simulink model "celp_sq"  (Simulink 6.1)
settings: Solver=FixedStepDiscrete  SolverMode=SingleTasking  StartTime=0.0  StopTime=3  RelTol=1e-3
PreLoadFcn:
  | load lpcvocoder.mat;
undefined symbols (not defined in the file): jet, magnitude, poly2lsf
libraries: simulink x25, dspindex x17, dspcelplib x14, dsparch4 x12, dspquant2 x10, dspstat3 x10, dspsrcs4 x9, dspbuff3 x8, dspsigops x7, dspmtrx3 x6, dsplp x5, dspmathops x4
(part 2 of 2)

== system celp_sq/CELP Decoder/Subframe Synthesis/Formant Post Filter/Subsystem for ARMA Coefficients ==
  Lpc : Inport  Port=1  LatchInput=off
  Bandwidth Expansion : Subsystem  mask(Bandwidth Expansion){alpha=0.65}
      mask prompts: alpha "Bandwidth expansion factor:"
      mask help:
      | Generate autoregressive (AR) polynomial with bandwidth expanded relative to the bandwidth of the input AR polynomial.
      |
      | By reducing the radius of the roots in an autoregressive polynomial (i.e., scaling them towards the origin of the Z-plane), the bandwidth of the spectral peaks in the frequency response is expanded (flattened).  This operation is often referred to as "bandwidth expansion".
      |
      | Bandwidth expansion factor must be in the range [0,1], where 1.0 yields no changes to the roots of the polynomial.
      mask Help: web(dspbhelp);
      mask Display: fprintf('Bandwidth\nExpansion\n%g', alpha)
  Bandwidth Expansion1 : Subsystem  mask(Bandwidth Expansion){alpha=0.75}
      mask prompts: alpha "Bandwidth expansion factor:"
      mask help:
      | Generate autoregressive (AR) polynomial with bandwidth expanded relative to the bandwidth of the input AR polynomial.
      |
      | By reducing the radius of the roots in an autoregressive polynomial (i.e., scaling them towards the origin of the Z-plane), the bandwidth of the spectral peaks in the frequency response is expanded (flattened).  This operation is often referred to as "bandwidth expansion".
      |
      | Bandwidth expansion factor must be in the range [0,1], where 1.0 yields no changes to the roots of the polynomial.
      mask Help: web(dspbhelp);
      mask Display: fprintf('Bandwidth\nExpansion\n%g', alpha)
  FirCoef : Outport
  IirCoef : Outport  Port=2
  wires:
  Lpc/1 -> Bandwidth Expansion/1(In1), Bandwidth Expansion1/1(In1)
  Bandwidth Expansion1/1(Out1) -> IirCoef/1
  Bandwidth Expansion/1(Out1) -> FirCoef/1

== system celp_sq/CELP Decoder/Subframe Synthesis/Gain Scaling Unit/For Iterator Subsystem1 ==
  note: g(n)
  note: y(n)
  note: y(n)=g(n)+0.9375y(n-1)
      | with IC=1
  note: Computation of gain scaling factor for each sample of the subframe
  ScalarGain : Inport  Port=1  LatchInput=off
  Assignment : Assignment  ElementSrc=External  Rows=-1  ColumnSrc=External
  Constant1 : Constant  Orientation=down  Value=zeros(40,1)  VectorParams1D=off
  For Iterator : ForIterator  IterationLimit=40
  filter : dsparch4/Digital Filter  DialogController=dspDDGCreate  DialogControllerArgs=DataTag8  TypePopup=IIR (all poles)  IIRFiltStruct=Direct form II transposed  AllPoleFiltStruct=Direct form  FIRFiltStruct=Direct form  CoeffSource=Specify via dialog  NumCoeffs=[1 -.95]  DenCoeffs="[1   -0.9375]"  BiQuadCoeffs=[1 0.3 0.4 1 0.1 0.2]  LatticeCoeffs=[0.2 0.4]  denIgnore=on  FiltPerSampPopup=One filter per frame  IC=1  ICnum=0  ICden=0  roundingMode=Floor  overflowMode=off  ScaleValues=1  scaleValueFracLength=14  stageInFracLength=15  stageOutFracLength=15
  VectorGain : Outport
  wires:
  For Iterator/1 -> Assignment/3
  Assignment/1 -> VectorGain/1
  Constant1/1 -> Assignment/1
  ScalarGain/1 -> filter/1
  filter/1 -> Assignment/2

== system celp_sq/CELP Decoder/Subframe Synthesis/Reconstruction of  Speech Subframe/Harmonic Shaper ==
  inRes : Inport  Port=1  LatchInput=off
  Delay : Inport  Port=2  LatchInput=off
  Beta : Inport  Port=3  LatchInput=off
  1-bz^(-D)2 : Subsystem  TreatAsAtomicUnit=on
  Energy normalization : Subsystem
  Pitch Synthesis Filtering 1/(1-b.z^(-D))2 : dsparch4/Digital Filter  DialogController=dspDDGCreate  DialogControllerArgs=DataTag9  TypePopup=IIR (all poles)  IIRFiltStruct=Direct form II transposed  AllPoleFiltStruct=Direct form  FIRFiltStruct=Direct form  CoeffSource=Input port(s)  NumCoeffs=[1 -.95]  DenCoeffs=[1 0.1]  BiQuadCoeffs=[1 0.3 0.4 1 0.1 0.2]  LatticeCoeffs=[0.2 0.4]  denIgnore=on  FiltPerSampPopup=One filter per frame  IC=0  ICnum=0  ICden=0  roundingMode=Floor  overflowMode=off  ScaleValues=1  scaleValueFracLength=14  stageInFracLength=15  stageOutFracLength=15
  OutRes : Outport
  wires:
  Pitch Synthesis Filtering 1/(1-b.z^(-D))2/1 -> Energy normalization/2(SigNew)
  inRes/1 -> Energy normalization/1(SigOrg), Pitch Synthesis Filtering 1/(1-b.z^(-D))2/1
  1-bz^(-D)2/1(Polynom) -> Pitch Synthesis Filtering 1/(1-b.z^(-D))2/2
  Delay/1 -> 1-bz^(-D)2/1(D_buf_1based)
  Beta/1 -> 1-bz^(-D)2/2(beta)
  Energy normalization/1(SigNew2) -> OutRes/1  "res"

== system celp_sq/CELP Decoder/Subframe Synthesis/Reconstruction of  Speech Subframe/LP Synthesis Filter ==
  Residual : Inport  Port=1  LatchInput=off
  LSF : Inport  Port=2  LatchInput=off
  LPC to/from RC : dsplp/LPC to//from RC  conversion=LPC to RC  perr=off  stability=off  error=Replace it with 1
  LSF/LSP to LPC Conversion : dsplp/LSF//LSP to LPC Conversion  input=LSF in range (0 pi)
  Time-Varying  Synthesis Filter 1/A(z) : dsparch4/Digital Filter  DialogController=dspDDGCreate  DialogControllerArgs=DataTag10  TypePopup=IIR (all poles)  IIRFiltStruct=Direct form II transposed  AllPoleFiltStruct=Lattice AR  FIRFiltStruct=Direct form  CoeffSource=Input port(s)  NumCoeffs=[1 -.95]  DenCoeffs=[1 0.1]  BiQuadCoeffs=[1 0.3 0.4 1 0.1 0.2]  LatticeCoeffs=[0.2 0.4]  denIgnore=off  FiltPerSampPopup=One filter per frame  IC=0  ICnum=0  ICden=0  roundingMode=Floor  overflowMode=off  ScaleValues=1  scaleValueFracLength=14  stageInFracLength=15  stageOutFracLength=15
  Sig : Outport
  LPC : Outport  Port=2
  wires:
  LSF/LSP to LPC Conversion/1 -> LPC to/from RC/1, LPC/1
  LPC to/from RC/1 -> Time-Varying  Synthesis Filter 1/A(z)/2
  Residual/1 -> Time-Varying  Synthesis Filter 1/A(z)/1
  Time-Varying  Synthesis Filter 1/A(z)/1 -> Sig/1  "S(n)"
  LSF/1 -> LSF/LSP to LPC Conversion/1

== system celp_sq/CELP Decoder/Subframe Synthesis/Reconstruction of  Speech Subframe/Pitch synthesis ==
  PitchRes : Inport  Port=1  LatchInput=off
  Delay : Inport  Port=2  LatchInput=off
  Beta : Inport  Port=3  LatchInput=off
  1-bz^(-D) : Subsystem  TreatAsAtomicUnit=on
  Pitch synthesis Filter 1/(1-b.z^(-D)) : dsparch4/Digital Filter  DialogController=dspDDGCreate  DialogControllerArgs=DataTag11  TypePopup=IIR (all poles)  IIRFiltStruct=Direct form II transposed  AllPoleFiltStruct=Direct form  FIRFiltStruct=Direct form  CoeffSource=Input port(s)  NumCoeffs=[1 -.95]  DenCoeffs=[1 0.1]  BiQuadCoeffs=[1 0.3 0.4 1 0.1 0.2]  LatticeCoeffs=[0.2 0.4]  denIgnore=on  FiltPerSampPopup=One filter per frame  IC=0  ICnum=0  ICden=0  roundingMode=Floor  overflowMode=off  ScaleValues=1  scaleValueFracLength=14  stageInFracLength=15  stageOutFracLength=15
  LPRes : Outport
  wires:
  1-bz^(-D)/1(Polynom) -> Pitch synthesis Filter 1/(1-b.z^(-D))/2
  Delay/1 -> 1-bz^(-D)/1(D_buf_1based)
  Beta/1 -> 1-bz^(-D)/2(beta)
  PitchRes/1 -> Pitch synthesis Filter 1/(1-b.z^(-D))/1
  Pitch synthesis Filter 1/(1-b.z^(-D))/1 -> LPRes/1

== system celp_sq/CELP Decoder/Subframe Synthesis/Reconstruction of  Speech Subframe/Reconstruction of  Pitch Residual Signal ==
  4SignBit : Inport  Port=1  LatchInput=off
  4Position : Inport  Port=2  LatchInput=off
  FCBgain : Inport  Port=3  LatchInput=off
  Frame Status : FrameConversion  OutFrame=Sample based
  Frame Status1 : FrameConversion  OutFrame=Sample based
  Product4 : Product  OutDataTypeMode=double  SaturateOnIntegerOverflow=on
  replace 4 selected samples by their sign and set others to zero : Subsystem  TreatAsAtomicUnit=on
  qPitchRes : Outport
  wires:
  Frame Status/1 -> replace 4 selected samples by their sign and set others to zero/1(4SignBit)
  Frame Status1/1 -> replace 4 selected samples by their sign and set others to zero/2(4Position)
  replace 4 selected samples by their sign and set others to zero/1(newPitchRes) -> Product4/1
  4SignBit/1 -> Frame Status/1
  4Position/1 -> Frame Status1/1
  Product4/1 -> qPitchRes/1
  FCBgain/1 -> Product4/2

== system celp_sq/CELP Encoder/Frame Analysis/Classical LPC analysis/  ==
  note: In this subsystem, LPC analysis is performed on a speech signal with a
      |
      | frame size of 30 ms (240 samples). This signal has an overlap of 10 ms
      |
      | (80 samples). Each frame is windowed using a Hamming window and 10th order
      |
      | autocorrelation coefficients are found. Using the Levinson Durbin
      |
      | algorithm, 10th order LP coefficients are calculated from the
      |
      | autocorrelation coefficients. Finally, the LP coefficients are modified
      |
      | using a bandwidth expansion block.

== system celp_sq/CELP Encoder/Frame Analysis/Classical LPC analysis/Bandwidth Expansion ==
  In1 : Inport  Port=1  LatchInput=off
  Window Function : dspsigops/Window Function  DialogController=dspDDGCreate  DialogControllerArgs=DataTag14  winmode=Apply window to input  wintype=User defined  sampmode=Continuous  samptime=1  N=64  Rs=50  beta=10  winsamp=Symmetric  UserWindow=bwexpwin  OptParams=on  UserParams=alpha  dataType=double  isSigned=on  wordLen=16  udDataType=sfix(16)  fracBitsMode=Best precision  numFracBits=15  roundingMode=Floor  overflowMode=off
  Out1 : Outport
  wires:
  In1/1 -> Window Function/1
  Window Function/1 -> Out1/1

== system celp_sq/CELP Encoder/Frame Analysis/LSF Interpolation/  ==
  note: In this subsystem the LSFs are interpolated, in order to:
      |
      | 1.  Avoid rapid changes in the LP parameters (LSFs) between successive frames
      |
      | 2.  Specify the synthesis filter parameters for each subframe.

== system celp_sq/CELP Encoder/Frame Analysis/LSF Vector Quantization/  ==
  note: In this portion of the subsystems, the following operations occur:
      |
      |
      | 1. Linear prediction (LP) coefficients are converted to line spectral
      |
      |    frequencies (LSFs). After quantization and interpolation, the stability
      |
      |    of the LP synthesis filter can be guaranteed in the LSF domain without
      |
      |    additional computation.
      |
      |
      | 2. Weighting factors used in the LSF quantization are calculated using the
      |
      |    method proposed by Paliwal and Atal*. In this method, the weight
      |
      |    assigned to a given LSF is proportional to the spectral sensitivity and
      |
      |    the value of the spectral envelope at the current LSF.
      |
      | *[ K.K. Paliwal and B.S. Atal, "Efficient vector quantization of LPC
      |
      |    parameters at 24 bits/frame," J. Acoust. Soc. Am., vol. 87, p. S39, 1990]

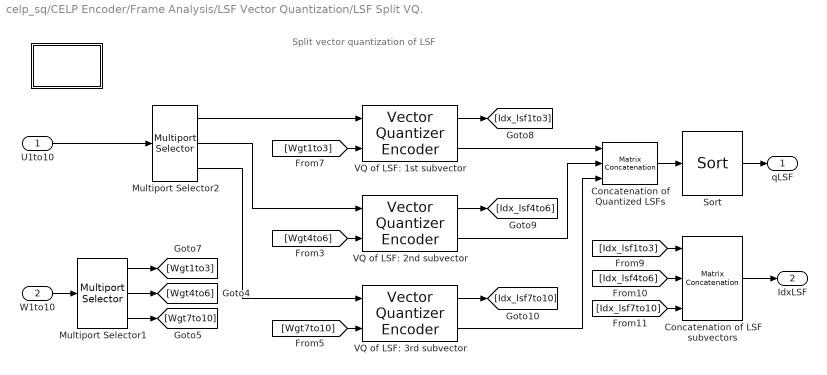
== system celp_sq/CELP Encoder/Frame Analysis/LSF Vector Quantization/LSF Split VQ. ==
  note: Split vector quantization of LSF
  U1to10 : Inport  Port=1  LatchInput=off
  W1to10 : Inport  Port=2  LatchInput=off
  " " : Subsystem
      mask Type: CELP Coder Demo Info
      mask Display: disp('Info')
  Concatenation of LSF subvectors : simulink/Math Operations/Matrix Concatenation  numInports=3  catMethod=Horizontal
  Concatenation of Quantized LSFs : simulink/Math Operations/Matrix Concatenation  numInports=3  catMethod=Vertical
  Multiport Selector1 : dspindex/Multiport Selector  rowsOrCols=Rows  idxCellArray={1:3,4:6,7:10}  idxErrMode=Clip Index
  Multiport Selector2 : dspindex/Multiport Selector  rowsOrCols=Rows  idxCellArray={1:3,4:6,7:10}  idxErrMode=Clip Index
  Sort : dspstat3/Sort  DialogController=dspDDGCreate  DialogControllerArgs=DataTag17  otype=Value  dir=Ascending  sortAlg=Quick sort  roundingMode=Floor  overflowMode=off
  VQ of LSF: 1st subvector : dspquant2/Vector Quantizer Encoder  CBsource=Specify via dialog  codebook=CB_lsf1to3_10bit  distMeasure=Weighted squared error  wgtSrc=Input port  weights=[1 1 1]  tieBreakRule=Choose the lower index  outQU=on  outQError=off  idtype=int32  roundingMode=Floor  overflowMode=off
  VQ of LSF: 2nd subvector : dspquant2/Vector Quantizer Encoder  CBsource=Specify via dialog  codebook=CB_lsf4to6_10bit  distMeasure=Weighted squared error  wgtSrc=Input port  weights=[1 1 1]  tieBreakRule=Choose the lower index  outQU=on  outQError=off  idtype=int32  roundingMode=Floor  overflowMode=off
  VQ of LSF: 3rd subvector : dspquant2/Vector Quantizer Encoder  CBsource=Specify via dialog  codebook=CB_lsf7to10_10bit  distMeasure=Weighted squared error  wgtSrc=Input port  weights=[1 1 1]  tieBreakRule=Choose the lower index  outQU=on  outQError=off  idtype=int32  roundingMode=Floor  overflowMode=off
  qLSF : Outport
  IdxLSF : Outport  Port=2
  wires:
  VQ of LSF: 1st subvector/2 -> Concatenation of Quantized LSFs/1
  VQ of LSF: 1st subvector/1 -> [Idx_lsf1to3]
  Multiport Selector2/2 -> VQ of LSF: 2nd subvector/1
  Multiport Selector2/3 -> VQ of LSF: 3rd subvector/1
  Multiport Selector1/2 -> [Wgt4to6]
  Multiport Selector1/3 -> [Wgt7to10]
  VQ of LSF: 2nd subvector/1 -> [Idx_lsf4to6]
  [Wgt7to10] -> VQ of LSF: 3rd subvector/2
  VQ of LSF: 3rd subvector/1 -> [Idx_lsf7to10]
  VQ of LSF: 2nd subvector/2 -> Concatenation of Quantized LSFs/2
  Concatenation of Quantized LSFs/1 -> Sort/1
  VQ of LSF: 3rd subvector/2 -> Concatenation of Quantized LSFs/3
  [Wgt4to6] -> VQ of LSF: 2nd subvector/2
  Multiport Selector1/1 -> [Wgt1to3]
  [Wgt1to3] -> VQ of LSF: 1st subvector/2
  [Idx_lsf1to3] -> Concatenation of LSF subvectors/1
  [Idx_lsf4to6] -> Concatenation of LSF subvectors/2
  [Idx_lsf7to10] -> Concatenation of LSF subvectors/3
  W1to10/1 -> Multiport Selector1/1
  U1to10/1 -> Multiport Selector2/1
  Sort/1 -> qLSF/1
  Concatenation of LSF subvectors/1 -> IdxLSF/1
  Multiport Selector2/1 -> VQ of LSF: 1st subvector/1

== system celp_sq/CELP Encoder/Frame Analysis/LSF Vector Quantization/Paliwal Weight  Computation ==
  note: Calculation of Perceptual Weighting Factors
  LSF : Inport  Port=1  LatchInput=off
  LPC : Inport  Port=2  LatchInput=off
  " " : Subsystem
      mask Type: CELP Coder Demo Info
      mask Display: disp('Info')
  Constant : Constant  Orientation=up  Value=0.15  VectorParams1D=off  SampleTime=-1
  Gain : Gain  Gain=-1
  Gain1 : Gain  Gain=[ones(1,8) 0.8 0.4]
  LPCpowSpec : Subsystem
  Math Function : Math  Operator=pow  SaturateOnIntegerOverflow=on
  Reshape : simulink/Math Operations/Reshape  OutputDimensionality=Column vector  OutputDimensions=[1,1]
  Submatrix : dspmtrx3/Submatrix  RowSpan=Range of rows  RowStartMode=Index  RowStartIndex=2  RowEndMode=Last  RowEndIndex=1  ColSpan=All columns  ColStartMode=First  ColStartIndex=1  ColEndMode=Last  ColEndIndex=1
  Weights : Outport
  wires:
  LPCpowSpec/1(Out) -> Math Function/1
  Constant/1 -> Math Function/2
  Math Function/1 -> Gain1/1
  Gain1/1 -> Reshape/1
  LSF/1 -> LPCpowSpec/2(LSF)
  Reshape/1 -> Weights/1
  Submatrix/1 -> Gain/1
  LPC/1 -> Submatrix/1
  Gain/1 -> LPCpowSpec/1(PC)

== system celp_sq/CELP Encoder/Subframe Analysis/Innovation signal quantization/  ==
  note: In this subsystem, the four "most significant pulses" are found from a
      |
      | subframe of length 40. Also, FCB gain is computed.
      |
      |
      |
      | 1. The absolute values of the 40 subframe samples are sorted in descending
      |
      | order. Their original positions are stored in a variable that has the
      |
      | following format: pos = [pos1, pos2, ..., pos40]. Here, pos1 stores the
      |
      | position of the largest valued sample, pos2 stores the position of the
      |
      | second largest valued sample, and so on.
      |
      |
      | 2.  The first four dominant samples are replaced by a +1 or a -1, where +1
      |
      | represents a positive sample and  -1 represents a negative sample. The
      |
      | other 36 samples are replaced by zeros. For example, a +1 or a -1 would be
      |
      | located at positions pos1, pos2, pos3, and pos4, and zeros would occupy the
      |
      | other positions.
      |
      |
      | 3. The zero-state response of the synthesis filter 1/A(z) to the original
      |
      | pitch residual signal is computed.
      |
      | 4. The zero-state response of the synthesis filter 1/A(z) to the quantized
      |
      | pitch residual signal is computed using the method of sparse filtering.
      |
      | Here, first the impulse response of the filter is calculated. Then the
      |
      | impulse response is convolved with the sparse representation of the
      |
      | quantized pitch residual signal.
      |
      |
      | 5. Steps 2 and 4 are repeated with four new samples from positions pos2,
      |
      | pos3, pos4, and pos5.
      |
      |
      |
      | This process is repeated for all 37 combinations of the positions. The set
      |
      | of four positions that minimize the error between the zero state response
      |
      | to the original pitch residual signal and the zero state response to the
      |
      | quantized pitch residual are the four "most significant pulses".

== system celp_sq/CELP Encoder/Subframe Analysis/Innovation signal quantization/Impulse Response ==
  In1 : Inport  Port=1  LatchInput=off
  DSP Constant : dspsrcs4/DSP Constant  Value=[1;zeros(39,1)]  SampleMode=Discrete  discreteOutput=Frame-based  continuousOutput=Sample-based  sampTime=1  framePeriod=-1  dataType=Inherit from 'Constant value'  isSigned=on  wordLen=16  udDataType=sfix(16)  fracBitsMode=Best precision  numFracBits=15  InterpretAs1D=-inf  Ts=-inf  FramebasedOutput=-inf
  For Iterator Subsystem2 : Subsystem  TreatAsAtomicUnit=on
      mask Display:
      | disp('Zero State\nIIR Lattice\nFilter');
      | port_label('input',1,'In');
      | port_label('input',2,'K');
      | port_label('output',1,'Out');
  Out1 : Outport
  wires:
  For Iterator Subsystem2/1(SigOut2) -> Out1/1
  In1/1 -> For Iterator Subsystem2/2(K)
  DSP Constant/1 -> For Iterator Subsystem2/1(SigIn2)

== system celp_sq/CELP Encoder/Subframe Analysis/Innovation signal quantization/Searching for FCB pulse  positions and FCB gain ==
  note: To Search for FCB pulse positions and FCB gain
  PitchRes : Inport  Port=1  LatchInput=off
  Idx : Inport  Port=2  LatchInput=off
  e_n : Inport  Port=3  LatchInput=off
  h : Inport  Port=4  LatchInput=off
  " " : Subsystem
      mask Type: CELP Coder Demo Info
      mask Display: disp('Info')
  1-based to  0-based : Bias  Bias=-1
  Computation of  Error and Gain : Subsystem
  For Iterator : ForIterator  ResetStates=reset  IterationLimit=37
  Optimal Features : Subsystem
  Partial decomposition of  Pitch Residual : Subsystem
  Signal to sign bit : Subsystem
  pos_sign_g : Outport
  wires:
  1-based to  0-based/1 -> Computation of  Error and Gain/2(4Pos)
  h/1 -> Computation of  Error and Gain/4(h)
  e_n/1 -> Computation of  Error and Gain/3(e_n)
  Signal to sign bit/1(SignBit) -> Computation of  Error and Gain/1(4Val), Optimal Features/1(SignBit)
  Partial decomposition of  Pitch Residual/2(4Idx) -> 1-based to  0-based/1, Optimal Features/4(Pos)
  Partial decomposition of  Pitch Residual/1(4Val) -> Signal to sign bit/1(Sig)
  For Iterator/1 -> Partial decomposition of  Pitch Residual/3(Control)
  Idx/1 -> Partial decomposition of  Pitch Residual/2(Idx)
  PitchRes/1 -> Partial decomposition of  Pitch Residual/1(PitchRes)
  Computation of  Error and Gain/1(Err) -> Optimal Features/2(Err)
  Computation of  Error and Gain/2(G) -> Optimal Features/3(G)
  Optimal Features/1(Features) -> pos_sign_g/1

== system celp_sq/CELP Encoder/Subframe Analysis/Innovation signal quantization/filter ==
  SigIn2 : Inport  Port=1  LatchInput=off
  K : Inport  Port=2  LatchInput=off
  " " : Subsystem
      mask Type: CELP Coder Demo Info
      mask Display: disp('Info')
  For Iterator : ForIterator  ResetStates=reset  IterationLimit=1  ShowIterationPort=off
  Time-Varying  Synthesis Filter 1/A(z). : dsparch4/Digital Filter  DialogController=dspDDGCreate  DialogControllerArgs=DataTag22  TypePopup=IIR (all poles)  IIRFiltStruct=Direct form II transposed  AllPoleFiltStruct=Lattice AR  FIRFiltStruct=Direct form  CoeffSource=Input port(s)  NumCoeffs=[1 -.95]  DenCoeffs=[1 0.1]  BiQuadCoeffs=[1 0.3 0.4 1 0.1 0.2]  LatticeCoeffs=[0.2 0.4]  denIgnore=off  FiltPerSampPopup=One filter per frame  IC=0  ICnum=0  ICden=0  roundingMode=Floor  overflowMode=off  ScaleValues=1  scaleValueFracLength=14  stageInFracLength=15  stageOutFracLength=15
  SigOut2 : Outport
  wires:
  Time-Varying  Synthesis Filter 1/A(z)./1 -> SigOut2/1
  SigIn2/1 -> Time-Varying  Synthesis Filter 1/A(z)./1
  K/1 -> Time-Varying  Synthesis Filter 1/A(z)./2

== system celp_sq/CELP Encoder/Subframe Analysis/Pitch Estimation/  ==
  note: Here the following operations occur:
      |
      | 1. The LPC residual signal is obtained by filtering the speech by the
      |     quantized and interpolated LPC analysis filter, A(Z).
      |
      | 2. The parameters specifying the adaptive component of the excitation
      |     (pitch lag and pitch gain) are computed using the open loop pitch estimation
      |     by minimizing the error between the current residual signal and its
      |     scaled-and-delayed version.

== system celp_sq/CELP Encoder/Subframe Analysis/Pitch Estimation/LPC Residual Calculation ==
  Speech : Inport  Port=1  LatchInput=off
  LSF : Inport  Port=2  LatchInput=off
  LPC to/from RC : dsplp/LPC to//from RC  conversion=LPC to RC  perr=off  stability=off  error=Replace it with 1
  LSF/LSP to LPC Conversion : dsplp/LSF//LSP to LPC Conversion  input=LSF in range (0 pi)
  Time-Varying  Analysis Filter A(z) : dsparch4/Digital Filter  DialogController=dspDDGCreate  DialogControllerArgs=DataTag23  TypePopup=FIR (all zeros)  IIRFiltStruct=Direct form II transposed  AllPoleFiltStruct=Direct form  FIRFiltStruct=Lattice MA  CoeffSource=Input port(s)  NumCoeffs=[1 -.95]  DenCoeffs=[1 0.1]  BiQuadCoeffs=[1 0.3 0.4 1 0.1 0.2]  LatticeCoeffs=[0.2 0.4]  denIgnore=on  FiltPerSampPopup=One filter per frame  IC=0  ICnum=0  ICden=0  roundingMode=Floor  overflowMode=off  ScaleValues=1  scaleValueFracLength=14  stageInFracLength=15  stageOutFracLength=15
  Residual : Outport
  K : Outport  Port=2
  wires:
  LSF/LSP to LPC Conversion/1 -> LPC to/from RC/1
  Speech/1 -> Time-Varying  Analysis Filter A(z)/1
  Time-Varying  Analysis Filter A(z)/1 -> Residual/1
  LSF/1 -> LSF/LSP to LPC Conversion/1
  LPC to/from RC/1 -> Time-Varying  Analysis Filter A(z)/2, K/1

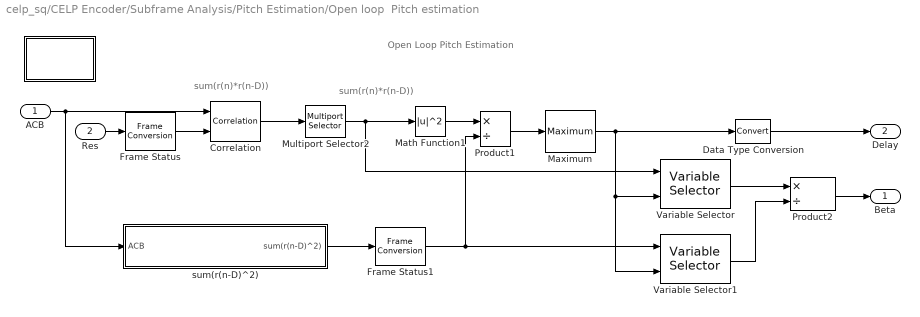
== system celp_sq/CELP Encoder/Subframe Analysis/Pitch Estimation/Open loop  Pitch estimation ==
  note: sum(r(n)*r(n-D))
  note: sum(r(n)*r(n-D))
  note: Open Loop Pitch Estimation
  ACB : Inport  Port=1  LatchInput=off
  Res : Inport  Port=2  LatchInput=off
  " " : Subsystem
      mask Type: CELP Coder Demo Info
      mask Display: disp('Info')
  Correlation : dspstat3/Correlation  DialogController=dspDDGCreate  DialogControllerArgs=DataTag24  domain=Fastest  roundingMode=Floor  overflowMode=off
  Data Type Conversion : DataTypeConversion  OutDataTypeMode=int32  SaturateOnIntegerOverflow=on  RndMeth=Zero
  Frame Status : FrameConversion  OutFrame=Sample based
  Frame Status1 : FrameConversion  OutFrame=Sample based
  Math Function1 : Math  Operator=magnitude^2  SaturateOnIntegerOverflow=on
  Maximum : dspstat3/Maximum  DialogController=dspDDGCreate  DialogControllerArgs=DataTag25  fcn=Index  reset=None  roundingMode=Floor  overflowMode=off
  Multiport Selector2 : dspindex/Multiport Selector  rowsOrCols=Rows  idxCellArray={40:167}  idxErrMode=Clip Index
  Product1 : Product  Inputs=*/  SaturateOnIntegerOverflow=on
  Product2 : Product  Inputs=*/  SaturateOnIntegerOverflow=on
  Variable Selector : dspindex/Variable Selector  rowsOrCols=Rows  IdxMode=Variable  Elements=[1 3]  ZerOneIdxMode=One-based  errmode=Generate Error
  Variable Selector1 : dspindex/Variable Selector  rowsOrCols=Rows  IdxMode=Variable  Elements=[1 3]  ZerOneIdxMode=One-based  errmode=Generate Error
  sum(r(n-D)^2) : Subsystem  TreatAsAtomicUnit=on
  Beta : Outport
  Delay : Outport  Port=2
  wires:
  Product2/1 -> Beta/1
  Variable Selector/1 -> Product2/1
  Maximum/1 -> Variable Selector1/2, Variable Selector/2, Data Type Conversion/1
  Product1/1 -> Maximum/1
  sum(r(n-D)^2)/1(sum(r(n-D)^2)) -> Frame Status1/1
  Math Function1/1 -> Product1/1
  Res/1 -> Frame Status/1
  ACB/1 -> Correlation/1, sum(r(n-D)^2)/1(ACB)
  Multiport Selector2/1 -> Variable Selector/1, Math Function1/1
  Correlation/1 -> Multiport Selector2/1
  Variable Selector1/1 -> Product2/2
  Frame Status/1 -> Correlation/2
  Frame Status1/1 -> Variable Selector1/1, Product1/2
  Data Type Conversion/1 -> Delay/1

== system celp_sq/CELP Encoder/Subframe Analysis/Pitch Estimation/Subframe Extraction ==
  Speech : Inport  Port=1  LatchInput=off
  LSF : Inport  Port=2  LatchInput=off
  SubFrIdx : Inport  Orientation=up  Port=3  LatchInput=off
  Frame to subframe : simulink/Math Operations/Reshape  OutputDimensionality=Customize  OutputDimensions=[40,4]
  Variable Selector : dspindex/Variable Selector  rowsOrCols=Columns  IdxMode=Variable  Elements=[1 3]  ZerOneIdxMode=One-based  errmode=Generate Error
  Variable Selector2 : dspindex/Variable Selector  rowsOrCols=Columns  IdxMode=Variable  Elements=[1 3]  ZerOneIdxMode=One-based  errmode=Generate Error
  Speech. : Outport
  LSF. : Outport  Port=2
  wires:
  SubFrIdx/1 -> Variable Selector/2, Variable Selector2/2
  Speech/1 -> Frame to subframe/1
  Variable Selector/1 -> Speech./1
  LSF/1 -> Variable Selector2/1
  Variable Selector2/1 -> LSF./1
  Frame to subframe/1 -> Variable Selector/1

== system celp_sq/CELP Encoder/Subframe Analysis/Pitch Residual computation/  ==
  note: In this portion of this subsystem, the following operations occur:
      |
      |
      | 1. Pitch gain is quantized using a 6-bit scalar quantizer
      |
      |
      | 2. Pitch delay, the integer-valued pitch lag (values within 1 to 128
      |
      |    inclusive), and the quantized value of pitch gain is used to form the
      |
      |    pitch residual signal. This pitch residual signal is defined as the
      |
      |    difference between the LPC residual signal and its scaled-and-delayed
      |
      |    version.

== system celp_sq/CELP Decoder/Subframe Synthesis/Formant Post Filter/Subsystem for ARMA Coefficients/Bandwidth Expansion ==
  In1 : Inport  Port=1  LatchInput=off
  Window Function : dspsigops/Window Function  DialogController=dspDDGCreate  DialogControllerArgs=DataTag4  winmode=Apply window to input  wintype=User defined  sampmode=Continuous  samptime=1  N=64  Rs=50  beta=10  winsamp=Symmetric  UserWindow=bwexpwin  OptParams=on  UserParams=alpha  dataType=double  isSigned=on  wordLen=16  udDataType=sfix(16)  fracBitsMode=Best precision  numFracBits=15  roundingMode=Floor  overflowMode=off
  Out1 : Outport
  wires:
  Window Function/1 -> Out1/1
  In1/1 -> Window Function/1

== system celp_sq/CELP Decoder/Subframe Synthesis/Formant Post Filter/Subsystem for ARMA Coefficients/Bandwidth Expansion1 ==
  In1 : Inport  Port=1  LatchInput=off
  Window Function : dspsigops/Window Function  DialogController=dspDDGCreate  DialogControllerArgs=DataTag5  winmode=Apply window to input  wintype=User defined  sampmode=Continuous  samptime=1  N=64  Rs=50  beta=10  winsamp=Symmetric  UserWindow=bwexpwin  OptParams=on  UserParams=alpha  dataType=double  isSigned=on  wordLen=16  udDataType=sfix(16)  fracBitsMode=Best precision  numFracBits=15  roundingMode=Floor  overflowMode=off
  Out1 : Outport
  wires:
  In1/1 -> Window Function/1
  Window Function/1 -> Out1/1

== system celp_sq/CELP Decoder/Subframe Synthesis/Reconstruction of  Speech Subframe/Harmonic Shaper/1-bz^(-D)2 ==
  note: 187-40+2 = 149
  D_buf_1based : Inport  Port=1  LatchInput=off
  beta : Inport  Port=2  LatchInput=off
  Assignment1 : Assignment  ElementSrc=External  Rows=-1  ColumnSrc=External
  DSP Constant : dspsrcs4/DSP Constant  Value=[1 zeros(1,187)]'  SampleMode=Discrete  discreteOutput=Frame-based  continuousOutput=Sample-based  sampTime=1  framePeriod=-1  dataType=double  isSigned=on  wordLen=16  udDataType=sfix(16)  fracBitsMode=Best precision  numFracBits=15  InterpretAs1D=-inf  Ts=-inf  FramebasedOutput=-inf
      settings: additionalParams=on
  DSP Constant1 : dspsrcs4/DSP Constant  Orientation=up  Value=149  SampleMode=Discrete  discreteOutput=Frame-based  continuousOutput=Sample-based  sampTime=-1  framePeriod=-1  dataType=Inherit from 'Constant value'  isSigned=on  wordLen=16  udDataType=sfix(16)  fracBitsMode=Best precision  numFracBits=15  InterpretAs1D=-inf  Ts=-inf  FramebasedOutput=-inf
  For Iterator : ForIterator  ResetStates=reset  IterationLimit=1  ShowIterationPort=off
  Frame Status1 : FrameConversion  OutFrame=Sample based
  Frame Status2 : FrameConversion  OutFrame=Sample based
  Gain : Gain  Gain=-0.965
  Sum3 : Sum  Inputs=|-+  SaturateOnIntegerOverflow=on
  Polynom : Outport
  wires:
  D_buf_1based/1 -> Sum3/1
  Frame Status2/1 -> Assignment1/3
  Gain/1 -> Assignment1/2
  Sum3/1 -> Frame Status2/1
  DSP Constant1/1 -> Sum3/2
  Frame Status1/1 -> Gain/1
  Assignment1/1 -> Polynom/1
  DSP Constant/1 -> Assignment1/1
  beta/1 -> Frame Status1/1

== system celp_sq/CELP Decoder/Subframe Synthesis/Reconstruction of  Speech Subframe/Harmonic Shaper/Energy normalization ==
  SigOrg : Inport  Port=1  LatchInput=off
  SigNew : Inport  Port=2  LatchInput=off
  DSP Constant : dspsrcs4/DSP Constant  Orientation=up  Value=eps  SampleMode=Discrete  discreteOutput=Frame-based  continuousOutput=Sample-based  sampTime=1  framePeriod=-1  dataType=Inherit from 'Constant value'  isSigned=on  wordLen=16  udDataType=sfix(16)  fracBitsMode=Best precision  numFracBits=15  InterpretAs1D=-inf  Ts=-inf  FramebasedOutput=-inf
  Math Function1 : Math  Operator=sqrt  SaturateOnIntegerOverflow=on
  Product1 : Product  Inputs=*/  SaturateOnIntegerOverflow=on
  Product2 : Product  SaturateOnIntegerOverflow=on
  Subsystem1 : Subsystem
      mask Display: disp('Energy\nCalculation')
  Subsystem2 : Subsystem
      mask Display: disp('Energy\nCalculation')
  Sum3 : Sum  Inputs=|++  SaturateOnIntegerOverflow=on
  SigNew2 : Outport
  wires:
  Product2/1 -> SigNew2/1
  SigOrg/1 -> Subsystem1/1(In1)
  SigNew/1 -> Product2/2, Subsystem2/1(In1)
  Math Function1/1 -> Product2/1
  Product1/1 -> Math Function1/1
  Subsystem1/1(Out1) -> Product1/1
  Sum3/1 -> Product1/2
  Subsystem2/1(Out1) -> Sum3/1
  DSP Constant/1 -> Sum3/2

== system celp_sq/CELP Decoder/Subframe Synthesis/Reconstruction of  Speech Subframe/Pitch synthesis/1-bz^(-D) ==
  D_buf_1based : Inport  Port=1  LatchInput=off
  beta : Inport  Port=2  LatchInput=off
  Assignment1 : Assignment  ElementSrc=External  Rows=-1  ColumnSrc=External
  DSP Constant : dspsrcs4/DSP Constant  Value=[1 zeros(1,187)]'  SampleMode=Discrete  discreteOutput=Frame-based  continuousOutput=Sample-based  sampTime=1  framePeriod=-1  dataType=double  isSigned=on  wordLen=16  udDataType=sfix(16)  fracBitsMode=Best precision  numFracBits=15  InterpretAs1D=-inf  Ts=-inf  FramebasedOutput=-inf
      settings: additionalParams=on
  DSP Constant1 : dspsrcs4/DSP Constant  Orientation=up  Value=149  SampleMode=Discrete  discreteOutput=Frame-based  continuousOutput=Sample-based  sampTime=-1  framePeriod=-1  dataType=int32  isSigned=on  wordLen=16  udDataType=sfix(16)  fracBitsMode=Best precision  numFracBits=15  InterpretAs1D=-inf  Ts=-inf  FramebasedOutput=-inf
      settings: additionalParams=on
  For Iterator : ForIterator  ResetStates=reset  IterationLimit=1  ShowIterationPort=off
  Frame Status : FrameConversion  OutFrame=Sample based
  Frame Status1 : FrameConversion  OutFrame=Sample based
  Gain : Gain  Gain=-1
  Sum3 : Sum  Inputs=|-+  SaturateOnIntegerOverflow=on
  Polynom : Outport
  wires:
  beta/1 -> Frame Status1/1
  DSP Constant/1 -> Assignment1/1
  Assignment1/1 -> Polynom/1
  Frame Status1/1 -> Gain/1
  DSP Constant1/1 -> Sum3/2
  Sum3/1 -> Frame Status/1
  Gain/1 -> Assignment1/2
  Frame Status/1 -> Assignment1/3
  D_buf_1based/1 -> Sum3/1

== system celp_sq/CELP Decoder/Subframe Synthesis/Reconstruction of  Speech Subframe/Reconstruction of  Pitch Residual Signal/replace 4 selected samples by their sign and set others to zero ==
  4SignBit : Inport  Port=1  LatchInput=off
  4Position : Inport  Port=2  LatchInput=off
  " " : Subsystem
      mask Type: CELP Coder Demo Info
      mask Display: disp('Info')
  For Iterator : ForIterator  ResetStates=reset  IterationLimit=1  ShowIterationPort=off
  Log all channels1 : dspcelplib/Log all channels  outType=Column vector  numRow=40  numCol=4  dType=int32
  newPitchRes : Outport
  wires:
  4SignBit/1 -> Log all channels1/1
  4Position/1 -> Log all channels1/2
  Log all channels1/1 -> newPitchRes/1

== system celp_sq/CELP Encoder/Frame Analysis/LSF Vector Quantization/LSF Split VQ./  ==
  note: In this subsystem, the LPC parameter vectors (LSFs) are quantized using a
      |
      | split vector quantization technique. This technique is a type of product-code
      |
      | vector quantization. In this method, a vector of ten LSFs (LSF1, LSF2, ..., LSF10)
      |
      | is divided into three subvectors. The first subvector contains the first
      |
      | three LSFs (LSF1, LSF2, LSF3). The second subvector contains the next three
      |
      | LSFs (LSF4, LSF5, LSF6). The third subvector contains the remaining four
      |
      | LSFs (LSF7, LSF8, LSF9, LSF10). Each of these subvectors is quantized
      |
      | separately using 10 bits.
      |
      |
      |
      |
      | The three codebooks that correspond to the three subvectors are generated
      |
      | using VQDTool from a training set of 200,000 LSF vectors using the
      |
      | Generalized Lloyd Algorithm (GLA). The weighted mean square error (WMSE)
      |
      | criterion is used as the distortion measure.
      |
      |
      |
      | In this subsystem, the best codebook entry for each subvector is selected
      |
      | based on the minimum weighted Euclidean distance measure. To arrive at the
      |
      | optimal codewords, a sequential search is conducted in each of the three
      |
      | codebooks. All three codewords are concatenated and sorted and thus
      |
      | ordering property in the quantized LSFs is ensured and the stability of the
      |
      | LP filter is guaranteed.

== system celp_sq/CELP Encoder/Frame Analysis/LSF Vector Quantization/Paliwal Weight  Computation/  ==
  note: Let the unquantized LSF vector is defined as LSF = [LSF1,LSF2, ...,LSF10].
      |
      |
      | The respective weighting vector is W = [w1, w2, ....,w8, 0.8*w9, 0.4*w10].
      |
      |
      | Within this weighting vector, the ith weighting factor, wi, is found using
      |
      | this equation [P(LSFi)]^1.5 (1<=i<=10), where P(f) is the LPC power
      |
      | spectrum associated with the LSF vector as a function of frequency, f].

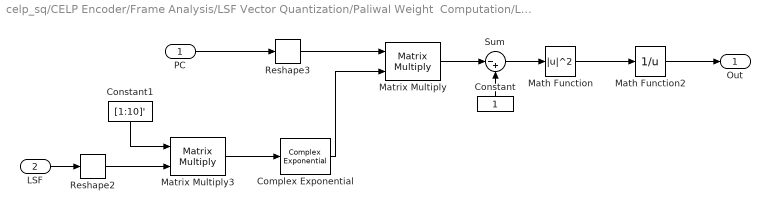
== system celp_sq/CELP Encoder/Frame Analysis/LSF Vector Quantization/Paliwal Weight  Computation/LPCpowSpec ==
  PC : Inport  Port=1  LatchInput=off
  LSF : Inport  Port=2  LatchInput=off
  Complex Exponential : dspmathops/Complex Exponential
  Constant : Constant  Orientation=up  VectorParams1D=off  SampleTime=-1
  Constant1 : Constant  Orientation=down  Value=[1:10]'  VectorParams1D=off  SampleTime=-1
  Math Function : Math  Operator=magnitude^2  SaturateOnIntegerOverflow=on
  Math Function2 : Math  Operator=reciprocal  SaturateOnIntegerOverflow=on
  Matrix Multiply : dspmtrx3/Matrix Multiply  numInputPorts=2  OptimizationLevel=None
  Matrix Multiply3 : dspmtrx3/Matrix Multiply  numInputPorts=2  OptimizationLevel=None
  Reshape2 : simulink/Math Operations/Reshape  OutputDimensionality=Row vector  OutputDimensions=[1,1]
  Reshape3 : simulink/Math Operations/Reshape  OutputDimensionality=Row vector  OutputDimensions=[1,1]
  Sum : Sum  Inputs=|-+  SaturateOnIntegerOverflow=on
  Out : Outport
  wires:
  Math Function2/1 -> Out/1
  Matrix Multiply/1 -> Sum/1
  PC/1 -> Reshape3/1
  Complex Exponential/1 -> Matrix Multiply/2
  Math Function/1 -> Math Function2/1
  Sum/1 -> Math Function/1
  Constant/1 -> Sum/2
  Reshape3/1 -> Matrix Multiply/1
  LSF/1 -> Reshape2/1
  Reshape2/1 -> Matrix Multiply3/2
  Constant1/1 -> Matrix Multiply3/1
  Matrix Multiply3/1 -> Complex Exponential/1

== system celp_sq/CELP Encoder/Subframe Analysis/Innovation signal quantization/Impulse Response/For Iterator Subsystem2 ==
  SigIn2 : Inport  Port=1  LatchInput=off
  K : Inport  Port=2  LatchInput=off
  For Iterator : ForIterator  ResetStates=reset  IterationLimit=1  ShowIterationPort=off
  Time-Varying  Synthesis Filter 1/A(z). : dsparch4/Digital Filter  DialogController=dspDDGCreate  DialogControllerArgs=DataTag18  TypePopup=IIR (all poles)  IIRFiltStruct=Direct form II transposed  AllPoleFiltStruct=Lattice AR  FIRFiltStruct=Direct form  CoeffSource=Input port(s)  NumCoeffs=[1 -.95]  DenCoeffs=[1 0.1]  BiQuadCoeffs=[1 0.3 0.4 1 0.1 0.2]  LatticeCoeffs=[0.2 0.4]  denIgnore=off  FiltPerSampPopup=One filter per frame  IC=0  ICnum=0  ICden=0  roundingMode=Floor  overflowMode=off  ScaleValues=1  scaleValueFracLength=14  stageInFracLength=15  stageOutFracLength=15
  SigOut2 : Outport
  wires:
  K/1 -> Time-Varying  Synthesis Filter 1/A(z)./2
  SigIn2/1 -> Time-Varying  Synthesis Filter 1/A(z)./1
  Time-Varying  Synthesis Filter 1/A(z)./1 -> SigOut2/1

== system celp_sq/CELP Encoder/Subframe Analysis/Innovation signal quantization/Searching for FCB pulse  positions and FCB gain/  ==
  note: This subsystem finds four FCB pulse positions and the
      | sign of the corresponding pulses based on the error between
      | the original pitch residual and its quantized version.

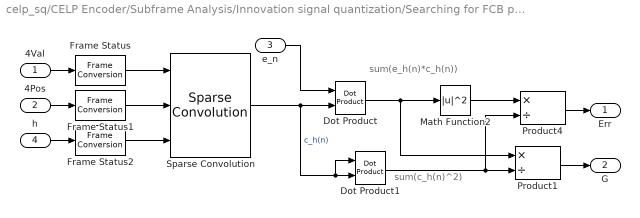
== system celp_sq/CELP Encoder/Subframe Analysis/Innovation signal quantization/Searching for FCB pulse  positions and FCB gain/Computation of  Error and Gain ==
  note: sum(e_h(n)*c_h(n))
  note: sum(c_h(n)^2)
  4Val : Inport  Port=1  LatchInput=off
  4Pos : Inport  Port=2  LatchInput=off
  e_n : Inport  Port=3  LatchInput=off
  h : Inport  Port=4  LatchInput=off
  Dot Product : simulink/Math Operations/Dot Product  OutDataType=sfix(16)  OutScaling=2^-10  DoSatur=on
  Dot Product1 : simulink/Math Operations/Dot Product  OutDataType=sfix(16)  OutScaling=2^-10  DoSatur=on
  Frame Status : FrameConversion
  Frame Status1 : FrameConversion
  Frame Status2 : FrameConversion
  Math Function2 : Math  Operator=magnitude^2  SaturateOnIntegerOverflow=on
  Product1 : Product  Inputs=*/  SaturateOnIntegerOverflow=on
  Product4 : Product  Inputs=*/  SaturateOnIntegerOverflow=on
  Sparse Convolution : dspcelplib/Sparse Convolution
  Err : Outport
  G : Outport  Port=2
  wires:
  Dot Product1/1 -> Product4/2, Product1/2
  Math Function2/1 -> Product4/1
  Dot Product/1 -> Math Function2/1, Product1/1
  Sparse Convolution/1 -> Dot Product/2, Dot Product1/2, Dot Product1/1  "c_h(n)"
  e_n/1 -> Dot Product/1
  4Val/1 -> Frame Status/1
  Product4/1 -> Err/1
  4Pos/1 -> Frame Status1/1
  h/1 -> Frame Status2/1
  Product1/1 -> G/1
  Frame Status/1 -> Sparse Convolution/1
  Frame Status1/1 -> Sparse Convolution/2
  Frame Status2/1 -> Sparse Convolution/3

== system celp_sq/CELP Encoder/Subframe Analysis/Innovation signal quantization/Searching for FCB pulse  positions and FCB gain/Optimal Features ==
  SignBit : Inport  Port=1  LatchInput=off
  Err : Inport  Port=2  LatchInput=off
  G : Inport  Port=3  LatchInput=off
  Pos : Inport  Port=4  LatchInput=off
  Data Type Conversion : DataTypeConversion  OutDataTypeMode=double  SaturateOnIntegerOverflow=on  RndMeth=Zero
  Data Type Conversion1 : DataTypeConversion  OutDataTypeMode=double  SaturateOnIntegerOverflow=on  RndMeth=Zero
  Delay1 : dspsigops/Delay  Orientation=left  dly_unit=Frames  delay=1  ic_detail=on  dif_ic_for_ch=off  dif_ic_for_dly=off  ic=0  reset_popup=None
  Feature  Concatenation : simulink/Math Operations/Matrix Concatenation  numInports=3  catMethod=Vertical
  Local maxima detector : Subsystem
  Switch : Switch  Criteria=u2 ~= 0  InputSameDT=on
  Features : Outport
  wires:
  Local maxima detector/1(Flag) -> Switch/2
  Switch/1 -> Delay1/1, Features/1
  Delay1/1 -> Switch/3
  Feature  Concatenation/1 -> Switch/1
  Data Type Conversion/1 -> Feature  Concatenation/1
  Data Type Conversion1/1 -> Feature  Concatenation/2
  Pos/1 -> Data Type Conversion/1
  SignBit/1 -> Data Type Conversion1/1
  G/1 -> Feature  Concatenation/3
  Err/1 -> Local maxima detector/1(Err)

== system celp_sq/CELP Encoder/Subframe Analysis/Innovation signal quantization/Searching for FCB pulse  positions and FCB gain/Partial decomposition of  Pitch Residual ==
  PitchRes : Inport  Port=1  LatchInput=off
  Idx : Inport  Port=2  LatchInput=off
  Control : Inport  Port=3  LatchInput=off
  Data Type Conversion : DataTypeConversion  OutDataTypeMode=double  SaturateOnIntegerOverflow=on  RndMeth=Zero
  Data Type Conversion1 : DataTypeConversion  OutDataTypeMode=int32  SaturateOnIntegerOverflow=on  RndMeth=Zero
  "Select Rows I, I+1, ...,I+3" : dspcelplib/Select Rows  numRows=4
  Sort : dspstat3/Sort  DialogController=dspDDGCreate  DialogControllerArgs=DataTag20  otype=Value  dir=Ascending  sortAlg=Quick sort  roundingMode=Floor  overflowMode=off
  Variable Selector1 : dspindex/Variable Selector  rowsOrCols=Rows  IdxMode=Variable  Elements=[1 3]  ZerOneIdxMode=One-based  errmode=Generate Error
  4Val : Outport
  4Idx : Outport  Port=2
  wires:
  Data Type Conversion1/1 -> 4Idx/1
  Idx/1 -> "Select Rows I, I+1, ...,I+3"/1
  Data Type Conversion/1 -> Sort/1
  "Select Rows I, I+1, ...,I+3"/1 -> Data Type Conversion/1
  Sort/1 -> Data Type Conversion1/1, Variable Selector1/2
  PitchRes/1 -> Variable Selector1/1
  Variable Selector1/1 -> 4Val/1
  Control/1 -> "Select Rows I, I+1, ...,I+3"/2

== system celp_sq/CELP Encoder/Subframe Analysis/Innovation signal quantization/Searching for FCB pulse  positions and FCB gain/Signal to sign bit ==
  Sig : Inport  Port=1  LatchInput=off
  Constant : Constant  Value=+1  OutDataTypeMode=int32
  Constant1 : Constant  Value=-1  OutDataTypeMode=int32
  Switch : Switch
  SignBit : Outport
  wires:
  Sig/1 -> Switch/2
  Constant1/1 -> Switch/3
  Constant/1 -> Switch/1
  Switch/1 -> SignBit/1

== system celp_sq/CELP Encoder/Subframe Analysis/Innovation signal quantization/filter/  ==
  note: This subsystem calculates the zero-state-reponse
      |
      | of the Time-Varying Synthesis Filter, 1/A(z),
      |
      | to the unquantized pitch residual signal.

== system celp_sq/CELP Encoder/Subframe Analysis/Pitch Estimation/Open loop  Pitch estimation/  ==
  note: In this subsystem, the pitch lag, D, and the optimal value of pitch gain,
      | beta, is computed. The current subframe of the residual signal is given by
      | [r(1) r(2) ... r(N)]. The mean squared error (MSE) between the current
      | subframe and the delayed-and-scaled version of this subframe (delay value,
      | D and scaling factor, beta) is given by E = sum(r(n) - beta*r(n-D)) where
      | this equation represents the summation over the whole subframe.
      |
      | The minimization of E over beta results in
      | beta = sum(r(n)*r(n-D))/ sum(r(n)*r(n)).
      |
      | The optimal beta is obtained when sum(r(n)*r(n-D))^2/ sum(r(n)*r(n))
      | is maximized.

== system celp_sq/CELP Encoder/Subframe Analysis/Pitch Estimation/Open loop  Pitch estimation/sum(r(n-D)^2) ==
  ACB : Inport  Port=1  LatchInput=off
  Autocorrelation : dspstat3/Autocorrelation  DialogController=dspDDGCreate  DialogControllerArgs=DataTag26  AllPositiveLags=off  maxlag=0  bias=None  domain=Time  roundingMode=Floor  overflowMode=off
  Constant : Constant  Orientation=up  Value=eps  VectorParams1D=off  SampleTime=-1
  For Iterator : ForIterator  IterationLimit=128
  Log all channels : dspcelplib/Log all channels  outType=Column vector  numRow=128  numCol=4  dType=double
  "Select Rows D, D+1,...D+39" : dspcelplib/Select Rows  numRows=40
  Sum3 : Sum  Inputs=|++  SaturateOnIntegerOverflow=on
  sum(r(n-D)^2) : Outport
  wires:
  Sum3/1 -> Log all channels/1
  Autocorrelation/1 -> Sum3/1
  Constant/1 -> Sum3/2
  Log all channels/1 -> sum(r(n-D)^2)/1
  [E1] -> Log all channels/2
  For Iterator/1 -> [E1], "Select Rows D, D+1,...D+39"/2  "r(n-D)"
  ACB/1 -> "Select Rows D, D+1,...D+39"/1
  "Select Rows D, D+1,...D+39"/1 -> Autocorrelation/1  "r(n-D)"

== system celp_sq/CELP Decoder/Subframe Synthesis/Reconstruction of  Speech Subframe/Harmonic Shaper/Energy normalization/Subsystem1 ==
  In1 : Inport  Port=1  LatchInput=off
  Dot Product : simulink/Math Operations/Dot Product  OutDataType=sfix(16)  OutScaling=2^-10  DoSatur=on
  Out1 : Outport
  wires:
  In1/1 -> Dot Product/1, Dot Product/2
  Dot Product/1 -> Out1/1

== system celp_sq/CELP Decoder/Subframe Synthesis/Reconstruction of  Speech Subframe/Harmonic Shaper/Energy normalization/Subsystem2 ==
  In1 : Inport  Port=1  LatchInput=off
  Dot Product : simulink/Math Operations/Dot Product  OutDataType=sfix(16)  OutScaling=2^-10  DoSatur=on
  Out1 : Outport
  wires:
  Dot Product/1 -> Out1/1
  In1/1 -> Dot Product/2, Dot Product/1

== system celp_sq/CELP Decoder/Subframe Synthesis/Reconstruction of  Speech Subframe/Reconstruction of  Pitch Residual Signal/replace 4 selected samples by their sign and set others to zero/  ==
  note: In this subsystem, the four samples whose positions are defined
      |
      | by the input position vector are replaced by a +1 or a -1 as determined
      |
      | by the input sign vector. The other 36 samples are replaced with zeros.

== system celp_sq/CELP Encoder/Subframe Analysis/Innovation signal quantization/Searching for FCB pulse  positions and FCB gain/Optimal Features/Local maxima detector ==
  note: Note: The 'Running Maximum' block
      | exploits the reset option in 'For' iterator
  Err : Inport  Port=1  LatchInput=off
  Relational Operator1 : RelationalOperator  Operator===  LogicOutDataTypeMode=Boolean  InputSameDT=on
  Running Maximum : dspstat3/Maximum  DialogController=dspDDGCreate  DialogControllerArgs=DataTag19  fcn=Running  reset=None  roundingMode=Floor  overflowMode=off
  Flag : Outport
  wires:
  Err/1 -> Running Maximum/1, Relational Operator1/1
  Running Maximum/1 -> Relational Operator1/2
  Relational Operator1/1 -> Flag/1
